simulink library "usask_tlm_lib"  (R2017b)
settings: Solver=ode45  StartTime=0.0  StopTime=10.0  RelTol=1e-3
undefined symbols (not defined in the file or in its folder): B, beta, d, K, L, lambda_1, m_E, m_G, mE_1, mE_2, mG_1, mG_2, nu, r1, r2, rho, T, Zc, Zc_1, Zc_2
libraries: usask_tlm_lib x6, transmission_lines x2
(part 2 of 4)

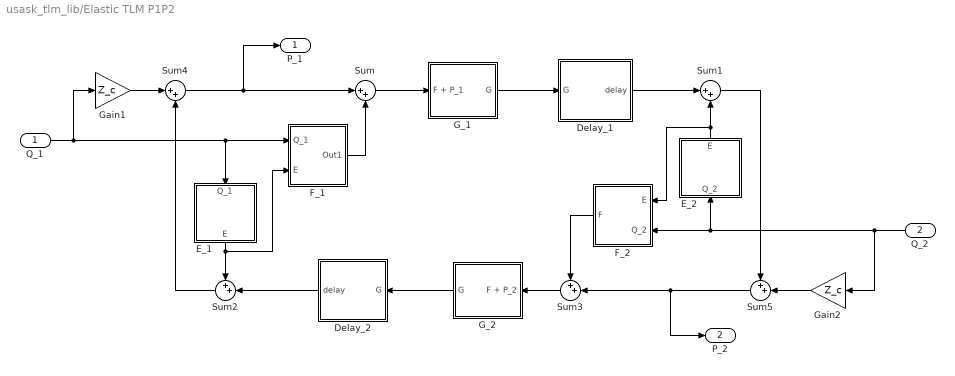
== system usask_tlm_lib/Elastic TLM P1P2 ==
  Q_1 : Inport
  Q_2 : Inport  Port=2
  "  Delay_2 " : Subsystem
      mask Display: disp('\fontname{Times New Roman}\ite^{-j\omegaT}', 'texmode', 'on')
  "Delay_1 " : Subsystem
      mask Display: disp('\fontname{Times New Roman}\ite^{-j\omegaT}', 'texmode', 'on')
  E_1 : Subsystem
      mask Display: disp('\fontname{Times New Roman}\fontsize{30}\itE', 'texmode', 'on')
  E_2 : Subsystem
      mask Display: disp('\fontname{Times New Roman}\fontsize{30}\itE', 'texmode', 'on')
  F_1 : Subsystem
      mask Display: disp('\fontname{Times New Roman}\fontsize{30}\itF', 'texmode', 'on')
  F_2 : Subsystem
      mask Display: disp('\fontname{Times New Roman}\fontsize{30}\itF', 'texmode', 'on')
  G_1 : Subsystem
      mask Display: disp('\fontname{Times New Roman}\fontsize{30}\itG', 'texmode', 'on')
  G_2 : Subsystem
      mask Display: disp('\fontname{Times New Roman}\fontsize{30}\itG', 'texmode', 'on')
  Gain1 : Gain  Gain=Z_c
  Gain2 : Gain  Gain=Z_c
  Sum : Sum  Inputs=|++
  Sum1 : Sum  Inputs=|++
  Sum2 : Sum  Inputs=++|
  Sum3 : Sum  Inputs=++|
  Sum4 : Sum  Inputs=|++
  Sum5 : Sum  Inputs=++|
  P_1 : Outport
  P_2 : Outport  Port=2
  wires:
  Sum/1 -> G_1/1(F + P_1)
  G_1/1(G) -> "Delay_1 "/1(G)
  E_2/1(E) -> Sum1/2, F_2/1(E)
  E_1/1(E) -> F_1/2(E), Sum2/1
  G_2/1(G) -> "  Delay_2 "/1(G)
  Q_1/1 -> Gain1/1, F_1/1(Q_1), E_1/1(Q_1)
  Sum4/1 -> P_1/1, Sum/1
  Sum3/1 -> G_2/1(F + P_2)
  F_2/1(F) -> Sum3/1
  Sum2/1 -> Sum4/2
  "Delay_1 "/1(delay) -> Sum1/1
  "  Delay_2 "/1(delay) -> Sum2/2
  Q_2/1 -> Gain2/1, F_2/2(Q_2), E_2/1(Q_2)
  Gain1/1 -> Sum4/1
  F_1/1(Out1) -> Sum/2
  Sum1/1 -> Sum5/1
  Gain2/1 -> Sum5/2
  Sum5/1 -> P_2/1, Sum3/2

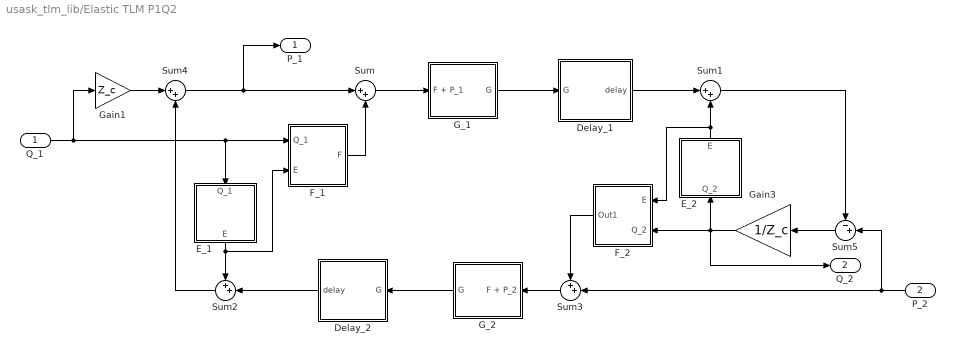
== system usask_tlm_lib/Elastic TLM P1Q2 ==
  Q_1 : Inport
  P_2 : Inport  Port=2
  "  Delay_2 " : Subsystem
      mask Display: disp('\fontname{Times New Roman}\ite^{-j\omegaT}', 'texmode', 'on')
  "Delay_1 " : Subsystem
      mask Display: disp('\fontname{Times New Roman}\ite^{-j\omegaT}', 'texmode', 'on')
  E_1 : Subsystem
      mask Display: disp('\fontname{Times New Roman}\fontsize{30}\itE', 'texmode', 'on')
  E_2 : Subsystem
      mask Display: disp('\fontname{Times New Roman}\fontsize{30}\itE', 'texmode', 'on')
  F_1 : Subsystem
      mask Display: disp('\fontname{Times New Roman}\fontsize{30}\itF', 'texmode', 'on')
  F_2 : Subsystem
      mask Display: disp('\fontname{Times New Roman}\fontsize{30}\itF', 'texmode', 'on')
  G_1 : Subsystem
      mask Display: disp('\fontname{Times New Roman}\fontsize{30}\itG', 'texmode', 'on')
  G_2 : Subsystem
      mask Display: disp('\fontname{Times New Roman}\fontsize{30}\itG', 'texmode', 'on')
  Gain1 : Gain  Gain=Z_c
  Gain3 : Gain  Gain=1/Z_c
  Sum : Sum  Inputs=|++
  Sum1 : Sum  Inputs=|++
  Sum2 : Sum  Inputs=++|
  Sum3 : Sum  Inputs=++|
  Sum4 : Sum  Inputs=|++
  Sum5 : Sum  Inputs=-+|
  P_1 : Outport
  Q_2 : Outport  Port=2
  wires:
  Sum/1 -> G_1/1(F + P_1)
  G_1/1(G) -> "Delay_1 "/1(G)
  E_2/1(E) -> Sum1/2, F_2/1(E)
  E_1/1(E) -> F_1/2(E), Sum2/1
  G_2/1(G) -> "  Delay_2 "/1(G)
  Q_1/1 -> Gain1/1, F_1/1(Q_1), E_1/1(Q_1)
  Sum4/1 -> P_1/1, Sum/1
  Sum3/1 -> G_2/1(F + P_2)
  F_2/1(Out1) -> Sum3/1
  Sum2/1 -> Sum4/2
  Sum1/1 -> Sum5/1
  P_2/1 -> Sum5/2, Sum3/2
  "Delay_1 "/1(delay) -> Sum1/1
  "  Delay_2 "/1(delay) -> Sum2/2
  Gain3/1 -> F_2/2(Q_2), E_2/1(Q_2), Q_2/1
  Gain1/1 -> Sum4/1
  Sum5/1 -> Gain3/1
  F_1/1(F) -> Sum/2

== system usask_tlm_lib/Elastic TLM Q1P2 ==
  P_1 : Inport
  Q_2 : Inport  Port=2
  "  Delay_2 " : Subsystem
      mask Display: disp('\fontname{Times New Roman}\ite^{-j\omegaT}', 'texmode', 'on')
  "Delay_1 " : Subsystem
      mask Display: disp('\fontname{Times New Roman}\ite^{-j\omegaT}', 'texmode', 'on')
  E_1 : Subsystem
      mask Display: disp('\fontname{Times New Roman}\fontsize{30}\itE', 'texmode', 'on')
  E_2 : Subsystem
      mask Display: disp('\fontname{Times New Roman}\fontsize{30}\itE', 'texmode', 'on')
  F_1 : Subsystem
      mask Display: disp('\fontname{Times New Roman}\fontsize{30}\itF', 'texmode', 'on')
  F_2 : Subsystem
      mask Display: disp('\fontname{Times New Roman}\fontsize{30}\itF', 'texmode', 'on')
  G_1 : Subsystem
      mask Display: disp('\fontname{Times New Roman}\fontsize{30}\itG', 'texmode', 'on')
  G_2 : Subsystem
      mask Display: disp('\fontname{Times New Roman}\fontsize{30}\itG', 'texmode', 'on')
  Gain1 : Gain  Gain=Z_c
  Gain2 : Gain  Gain=1/Z_c
  Sum : Sum  Inputs=|++
  Sum1 : Sum  Inputs=|++
  Sum2 : Sum  Inputs=++|
  Sum3 : Sum  Inputs=++|
  Sum4 : Sum  Inputs=++|
  Sum6 : Sum  Inputs=|+-
  Q_1 : Outport
  P_2 : Outport  Port=2
  wires:
  Sum/1 -> G_1/1(F + P_1)
  G_1/1(G) -> "Delay_1 "/1(G)
  E_2/1(E) -> Sum1/2, F_2/1(E)
  E_1/1(E) -> F_1/2(E), Sum2/1
  G_2/1(G) -> "  Delay_2 "/1(G)
  P_1/1 -> Sum6/1, Sum/1
  Sum3/1 -> G_2/1(F + P_2)
  F_2/1(Out1) -> Sum3/1
  "Delay_1 "/1(delay) -> Sum1/1
  "  Delay_2 "/1(delay) -> Sum2/2
  Q_2/1 -> Gain1/1, F_2/2(Q_2), E_2/1(Q_2)
  F_1/1(F) -> Sum/2
  Sum6/1 -> Gain2/1
  Gain2/1 -> Q_1/1, F_1/1(Q_1), E_1/1(Q_1)
  Sum2/1 -> Sum6/2
  Sum1/1 -> Sum4/1
  Sum4/1 -> P_2/1, Sum3/2
  Gain1/1 -> Sum4/2

== system usask_tlm_lib/Elastic TLM Q1Q2 ==
  P_1 : Inport
  P_2 : Inport  Port=2
  "  Delay_2 " : Subsystem
      mask Display: disp('\fontname{Times New Roman}\ite^{-j\omegaT}', 'texmode', 'on')
  "Delay_1 " : Subsystem
      mask Display: disp('\fontname{Times New Roman}\ite^{-j\omegaT}', 'texmode', 'on')
  E_1 : Subsystem
      mask Display: disp('\fontname{Times New Roman}\fontsize{30}\itE', 'texmode', 'on')
  E_2 : Subsystem
      mask Display: disp('\fontname{Times New Roman}\fontsize{30}\itE', 'texmode', 'on')
  F_1 : Subsystem
      mask Display: disp('\fontname{Times New Roman}\fontsize{30}\itF', 'texmode', 'on')
  F_2 : Subsystem
      mask Display: disp('\fontname{Times New Roman}\fontsize{30}\itF', 'texmode', 'on')
  G_1 : Subsystem
      mask Display: disp('\fontname{Times New Roman}\fontsize{30}\itG', 'texmode', 'on')
  G_2 : Subsystem
      mask Display: disp('\fontname{Times New Roman}\fontsize{30}\itG', 'texmode', 'on')
  Gain2 : Gain  Gain=1/Z_c
  Gain3 : Gain  Gain=1/Z_c
  Sum : Sum  Inputs=|++
  Sum1 : Sum  Inputs=|++
  Sum2 : Sum  Inputs=++|
  Sum3 : Sum  Inputs=++|
  Sum5 : Sum  Inputs=-+|
  Sum6 : Sum  Inputs=|+-
  Q_1 : Outport
  Q_2 : Outport  Port=2
  wires:
  Sum/1 -> G_1/1(F + P_1)
  G_1/1(G) -> "Delay_1 "/1(G)
  E_2/1(E) -> Sum1/2, F_2/1(E)
  E_1/1(E) -> F_1/2(E), Sum2/1
  G_2/1(G) -> "  Delay_2 "/1(G)
  Sum3/1 -> G_2/1(F + P_2)
  F_2/1(F) -> Sum3/1
  Sum1/1 -> Sum5/1
  P_2/1 -> Sum5/2, Sum3/2
  "Delay_1 "/1(delay) -> Sum1/1
  "  Delay_2 "/1(delay) -> Sum2/2
  Gain3/1 -> F_2/2(Q_2), E_2/1(Q_2), Q_2/1
  Sum5/1 -> Gain3/1
  F_1/1(F) -> Sum/2
  P_1/1 -> Sum6/1, Sum/1
  Sum6/1 -> Gain2/1
  Gain2/1 -> Q_1/1, F_1/1(Q_1), E_1/1(Q_1)
  Sum2/1 -> Sum6/2

== system usask_tlm_lib/Internal Blocks ==
  Tapered TLM Base : Subsystem  mask(Tapered Hydraulic Transmission Line (TLM)){Zc_1=Zc_1, Zc_2=Zc_2, beta=beta, T=T, lambda_1=lambda_1}
      mask help:
      | This model implements the transmission line model in Wiens and ven der Buhs (2018).
      |
      | This model assumes laminar flow in a rigid-walled tube with a linear taper in radius between the two ports. It assumes constant bulk modulus (no cavitation or entrined air effects) and includes frequency-dependent friction effects.
      |
      | Positive flows are directed into either port.
      |
      | This model also assumes zero initial conditions
      |
      | Reference:
      | Travis Wiens and Jeremy vsn der Buhs. In Improved Transmission Line Model for Dynamic Laminar Flow Through Tapered Tubes. Proceedings of the Bath/ASME Symposium on Fluid Power and Motion Control, Bath, 2018
      mask init:
      | lambda_2=1/lambda_1;
      | 
      | R=Zc_1*beta*8*(3/(1+lambda_1+lambda_1^2));%laminar resistance
      | 
      | k=6; % Number of weighting factors
      | 
      | % Grab optimized weighting factors and parameters. Please see paper for
      | % more detail on how these parameters were found.
      | [ mE_1, mG_1, tau_1, K_diff1, K_mean1 ] = interpolateTLMparamsFIR( beta, lambda_1, k);
      | [ mE_2, mG_2, tau_2, K_diff2, K_mean2 ] = interpolateTLMparamsFIR( beta, lambda_2, k);
      | 
      | %Todo: fix error checkings
      | % if isnan(mE_1(1)) || isnan(mG_1(1)) || isnan(tau_1) ||isnan(mE_2(1)) || isnan(mG_2(1)) || isnan(tau_2)
      | %     error('The parameters you have entered are outside the working range of this model. Weighting factors cannot be found')
      | % end
      | 
      | T_1 = tau_1*T; % Modified wave propagation time (s), Equation (18)
      | T_2 = tau_2*T; % Modified wave propagation time (s), Equation (18)
      | 
      | n=nan(1,k); % Weighting factor initialization
      | n(1)=0.3/(1+3*beta);
      | for i=2:k
      |     n(i)=n(i-1)*3; 
      | end
      | 
      | % H 
      | H_1DC=K_mean1*(1/lambda_1.^2 -1)/(8*beta*3/(1+lambda_1+lambda_1^2)+1/lambda_1^2+1);
      | H_2DC=K_mean2*(1/lambda_2.^2 -1)/(8*beta*3/(1+lambda_2+lambda_2^2)+1/lambda_2^2+1);
      | 
      | H_1mean=H_1DC/(2*T_1);
      | H_2mean=H_2DC/(2*T_2);
      | 
      | H_1a=K_diff1*H_1mean;
      | H_1b=(2-K_diff1)*H_1mean;
      | 
      | H_2a=K_diff2*H_2mean;
      | H_2b=(2-K_diff2)*H_2mean;
      | 
      | 
      | % E
      | E_1DC=Zc_1*sum(mE_1./n);
      | E_2DC=Zc_2*sum(mE_2./n);
      | 
      | b_1=1-8*beta/(E_1DC/Zc_1);
      | b_2=1-8*beta/(E_2DC/Zc_2);
      | 
      | % F
      | F_1DC=Zc_1+b_1*E_1DC;
      | F_2DC=Zc_2+b_2*E_2DC;
      | 
      | F_k1=((1-H_1DC)*(E_2DC+Zc_2-R)+H_2DC*(E_1DC+Zc_1))/(1-H_1DC-H_2DC)/F_1DC
      | F_k2=((1-H_2DC)*(E_1DC+Zc_1-R)+H_1DC*(E_2DC+Zc_2))/(1-H_2DC-H_1DC)/F_2DC
      | 
      | %Error Checking
      | % load TaperedTLMAcceptableErrorContour.mat
      | % IN = inpolygon(lambda_1,beta,lambda_poly,beta_poly);
      | % if ~IN
      | %     warning('Dissipaton number (beta) and taper ratio (lambda) combination are outside the recommended range')
      | % end
      | %warning('need to reinstate polygon error checking')
      | 
      | 
      | 
      | 
      | %% End of initialization
      mask DialogControl DescGroupVar Prompt: Tapered Hydraulic Transmission Line (TLM)
  Tapered TLM Segment : Subsystem  mask(Tapered Hydraulic Transmission Line (TLM)){Zc_1=Zc(2), Zc_2=Zc(3), beta=beta(2), T=T(2), lambda_1=lambda_1(2)}
      mask help:
      | This model implements the transmission line model in Wiens and ven der Buhs (2018).
      |
      | This model assumes a rigid-walled tube with a linear taper in radius between the two ports. It assumes constant bulk modulus (no cavitation or entrined air effects) and includes frequency-dependent friction effects.
      |
      | Positive flows are directed into either port.
      |
      | This model also assumes zero initial conditions
      |
      | Reference:
      | Travis Wiens and Jeremy vsn der Buhs. In Improved Transmission Line Model for Dynamic Laminar Flow Through Tapered Tubes. Proceedings of the Bath/ASME Symposium on Fluid Power and Motion Control, Bath, 2018
      mask init:
      | lambda_2=1/lambda_1;
      | 
      | R=Zc_1*beta*8*(3/(1+lambda_1+lambda_1^2));%laminar resistance
      | 
      | k=6; % Number of weighting factors
      | 
      | % Grab optimized weighting factors and parameters. Please see paper for
      | % more detail on how these parameters were found.
      | [ mE_1, mG_1, tau_1, K_diff1, K_mean1 ] = interpolateTLMparamsFIR( beta, lambda_1, k);
      | [ mE_2, mG_2, tau_2, K_diff2, K_mean2 ] = interpolateTLMparamsFIR( beta, lambda_2, k);
      | 
      | %Todo: fix error checkings
      | % if isnan(mE_1(1)) || isnan(mG_1(1)) || isnan(tau_1) ||isnan(mE_2(1)) || isnan(mG_2(1)) || isnan(tau_2)
      | %     error('The parameters you have entered are outside the working range of this model. Weighting factors cannot be found')
      | % end
      | 
      | T_1 = tau_1*T; % Modified wave propagation time (s), Equation (18)
      | T_2 = tau_2*T; % Modified wave propagation time (s), Equation (18)
      | 
      | n=nan(1,k); % Weighting factor initialization
      | n(1)=0.3/(1+3*beta);
      | for i=2:k
      |     n(i)=n(i-1)*3; 
      | end
      | 
      | % H 
      | H_1DC=K_mean1*(1/lambda_1.^2 -1)/(8*beta*3/(1+lambda_1+lambda_1^2)+1/lambda_1^2+1);
      | H_2DC=K_mean2*(1/lambda_2.^2 -1)/(8*beta*3/(1+lambda_2+lambda_2^2)+1/lambda_2^2+1);
      | 
      | C_1mean=H_1DC/(2*T_1);
      | C_2mean=H_2DC/(2*T_2);
      | 
      | % C_1mean=H_1DC;
      | % C_2mean=H_2DC;
      | 
      | H_1a=K_diff1*C_1mean;
      | H_1b=(2-K_diff1)*C_1mean;
      | 
      | H_2a=K_diff2*C_2mean;
      | H_2b=(2-K_diff2)*C_2mean;
      | 
      | 
      | %N_H=100;%make this a parameter
      | 
      | %H_1=[linspace(H_1a,H_1b,N_H)]*(2*T_1)./(N_H);
      | %H_2=[linspace(H_2a,H_2b,N_H)]*(2*T_2)./(N_H);
      | 
      | % E
      | E_1DC=Zc_1*sum(mE_1./n);
      | E_2DC=Zc_2*sum(mE_2./n);
      | 
      | b_1=1-8*beta/(E_1DC/Zc_1);% eq (16)
      | b_2=1-8*beta/(E_2DC/Zc_2);% eq (16)
      | 
      | % F
      | F_1DC=Zc_1+b_1*E_1DC;
      | F_2DC=Zc_2+b_2*E_2DC;
      | 
      | F_k1=((1-H_1DC)*(E_2DC+Zc_2-R)+H_2DC*(E_1DC+Zc_1))/(1-H_1DC-H_2DC)/F_1DC
      | F_k2=((1-H_2DC)*(E_1DC+Zc_1-R)+H_1DC*(E_2DC+Zc_2))/(1-H_2DC-H_1DC)/F_2DC
      | 
      | %Error Checking
      | % load TaperedTLMAcceptableErrorContour.mat
      | % IN = inpolygon(lambda_1,beta,lambda_poly,beta_poly);
      | % if ~IN
      | %     warning('Dissipaton number (beta) and taper ratio (lambda) combination are outside the recommended range')
      | % end
      | warning('need to reinstate polygon error checking')
      | 
      | 
      | 
      | 
      | %% End of initialization
      mask DialogControl DescGroupVar Prompt: Tapered Hydraulic Transmission Line (TLM)

== system usask_tlm_lib/TLM Johnston P1P2 ==
  Q1 : Inport
  Q2 : Inport  Port=2
  E1 : transmission_lines/TLM Krus P1P2/E1
  E2 : Subsystem
  F1 : transmission_lines/TLM Krus P1P2/F1
  F2 : Subsystem
  G1 : Subsystem
  G2 : Subsystem
  Gain : Gain  Gain=Zc
  Gain1 : Gain  Gain=Zc
  Sum : Sum  Inputs=|++
  Sum1 : Sum  Inputs=++|
  Sum2 : Sum  Inputs=++|
  Sum3 : Sum  Inputs=|++
  Sum4 : Sum  Inputs=|++
  Sum5 : Sum  Inputs=++|
  Transport Delay1 : TransportDelay  DelayTime=T
  Transport Delay2 : TransportDelay  DelayTime=T
  P1 : Outport
  P2 : Outport  Port=2
  wires:
  Sum3/1 -> Sum5/1  "C2"
  G1/1(Out) -> Transport Delay1/1
  E2/1(Out) -> Sum3/2
  Sum5/1 -> Sum2/2, P2/1  "P2"
  Sum2/1 -> G2/1(In)
  F2/1(Out) -> Sum2/1
  Q2/1 -> F2/1(In), E2/1(In), Gain1/1  "Q2"
  Transport Delay1/1 -> Sum3/1
  Gain1/1 -> Sum5/2
  Sum/1 -> G1/1(In)
  Transport Delay2/1 -> Sum1/2
  Sum1/1 -> Sum4/1  "C1"
  F1/1 -> Sum/2
  E1/1 -> Sum1/1
  G2/1(Out) -> Transport Delay2/1
  Q1/1 -> Gain/1, F1/1, E1/1  "Q1"
  Sum4/1 -> P1/1, Sum/1  "P1"
  Gain/1 -> Sum4/2

== system usask_tlm_lib/TLM Johnston P1Q2 ==
  Q1 : Inport
  P2 : Inport  Port=2
  Ea : Subsystem
  Eb : Subsystem
  Fa : Subsystem
  Fb : Subsystem
  Ga : Subsystem
  Gain : Gain  Gain=Zc
  Gain1 : Gain  Gain=1/Zc
  Gb : Subsystem
  Sum : Sum  Inputs=|++
  Sum1 : Sum  Inputs=++|
  Sum2 : Sum  Inputs=++|
  Sum3 : Sum  Inputs=|++
  Sum4 : Sum  Inputs=|++
  Sum5 : Sum  Inputs=-+|
  Transport Delay1 : TransportDelay  DelayTime=T
  Transport Delay2 : TransportDelay  DelayTime=T
  P1 : Outport
  Q2 : Outport  Port=2
  wires:
  Sum4/1 -> P1/1, Sum/1  "P1"
  Sum/1 -> Ga/1(In)
  Transport Delay2/1 -> Sum3/1
  Gain/1 -> Sum4/1
  Sum5/1 -> Gain1/1
  Transport Delay1/1 -> Sum1/2
  Q1/1 -> Gain/1, Ea/1(In), Fa/1(In)
  Sum1/1 -> Sum4/2
  Fa/1(Out) -> Sum/2
  Gain1/1 -> Q2/1, Eb/1(In), Fb/1(In)  "Q2"
  Fb/1(Out) -> Sum2/1
  Sum2/1 -> Gb/1(In)
  Ea/1(Out) -> Sum1/1
  Gb/1(Out) -> Transport Delay1/1
  P2/1 -> Sum5/2, Sum2/2
  Eb/1(Out) -> Sum3/2
  Ga/1(Out) -> Transport Delay2/1
  Sum3/1 -> Sum5/1  "C2"

== system usask_tlm_lib/TLM Johnston Q1P2 ==
  P1 : Inport
  Q2 : Inport  Port=2
  Ea : Subsystem
  Eb : Subsystem
  Fa : Subsystem
  Fb : Subsystem
  Ga : Subsystem
  Gain : Gain  Gain=1/Zc
  Gain1 : Gain  Gain=Zc
  Gb : Subsystem
  Sum : Sum  Inputs=|++
  Sum1 : Sum  Inputs=++|
  Sum2 : Sum  Inputs=++|
  Sum3 : Sum  Inputs=|++
  Sum4 : Sum  Inputs=|+-
  Sum5 : Sum  Inputs=++|
  Transport Delay1 : TransportDelay  DelayTime=T
  Transport Delay2 : TransportDelay  DelayTime=T
  Q1 : Outport
  P2 : Outport  Port=2
  wires:
  Gain1/1 -> Sum5/2
  P1/1 -> Sum4/1, Sum/1  "P1"
  Sum/1 -> Ga/1(In)
  Transport Delay2/1 -> Sum3/1
  Transport Delay1/1 -> Sum1/2
  Gain/1 -> Q1/1, Ea/1(In), Fa/1(In)  "Q1"
  Sum1/1 -> Sum4/2  "C1"
  Fa/1(Out) -> Sum/2
  Q2/1 -> Gain1/1, Eb/1(In), Fb/1(In)  "Q2"
  Fb/1(Out) -> Sum2/1
  Sum2/1 -> Gb/1(In)
  Ea/1(Out) -> Sum1/1
  Gb/1(Out) -> Transport Delay1/1
  Sum5/1 -> P2/1, Sum2/2  "P2"
  Eb/1(Out) -> Sum3/2
  Ga/1(Out) -> Transport Delay2/1
  Sum3/1 -> Sum5/1  "C2"
  Sum4/1 -> Gain/1

== system usask_tlm_lib/TLM Johnston Q1Q2 ==
  P1 : Inport
  P2 : Inport  Port=2
  Ea : Subsystem
  Eb : Subsystem
  Fa : Subsystem
  Fb : Subsystem
  Ga : Subsystem
  Gain : Gain  Gain=1/Zc
  Gain1 : Gain  Gain=1/Zc
  Gb : Subsystem
  Sum : Sum  Inputs=|++
  Sum1 : Sum  Inputs=++|
  Sum2 : Sum  Inputs=++|
  Sum3 : Sum  Inputs=|++
  Sum4 : Sum  Inputs=|+-
  Sum5 : Sum  Inputs=-+|
  Transport Delay1 : TransportDelay  DelayTime=T
  Transport Delay2 : TransportDelay  DelayTime=T
  Q1 : Outport
  Q2 : Outport  Port=2
  wires:
  P1/1 -> Sum4/1, Sum/1  "P1"
  Sum/1 -> Ga/1(In)
  Transport Delay2/1 -> Sum3/1
  Sum5/1 -> Gain1/1
  Transport Delay1/1 -> Sum1/2
  Gain/1 -> Q1/1, Ea/1(In), Fa/1(In)  "Q1"
  Sum1/1 -> Sum4/2  "C1"
  Fa/1(Out) -> Sum/2
  Gain1/1 -> Q2/1, Eb/1(In), Fb/1(In)  "Q2"
  Fb/1(Out) -> Sum2/1
  Sum2/1 -> Gb/1(In)
  Ea/1(Out) -> Sum1/1
  Gb/1(Out) -> Transport Delay1/1
  P2/1 -> Sum5/2, Sum2/2
  Eb/1(Out) -> Sum3/2
  Ga/1(Out) -> Transport Delay2/1
  Sum3/1 -> Sum5/1  "C2"
  Sum4/1 -> Gain/1

== system usask_tlm_lib/TLM Krus P1P2 ==
  Q1 : Inport
  Q2 : Inport  Port=2
  E1 : Subsystem
  E2 : Subsystem
  F1 : Subsystem
  F2 : Subsystem
  G1 : Subsystem
  G2 : Subsystem
  Gain : Gain  Gain=Zc
  Gain1 : Gain  Gain=Zc
  Sum : Sum  Inputs=|++
  Sum1 : Sum  Inputs=++|
  Sum2 : Sum  Inputs=++|
  Sum3 : Sum  Inputs=|++
  Sum4 : Sum  Inputs=|++
  Sum5 : Sum  Inputs=++|
  Transport Delay1 : TransportDelay  DelayTime=T
  Transport Delay2 : TransportDelay  DelayTime=T
  P1 : Outport
  P2 : Outport  Port=2
  wires:
  Gain/1 -> Sum4/2
  Sum4/1 -> Sum/1, P1/1  "P1"
  Q1/1 -> E1/1(In), F1/1(In), Gain/1  "Q1"
  Sum3/1 -> Sum5/1  "C2"
  Sum5/1 -> P2/1, Sum2/2  "P2"
  Q2/1 -> E2/1(In), F2/1(In), Gain1/1  "Q2"
  Gain1/1 -> Sum5/2
  G1/1(Out) -> Transport Delay2/1
  E2/1(Out) -> Sum3/2
  G2/1(Out) -> Transport Delay1/1
  E1/1(Out) -> Sum1/1
  Sum2/1 -> G2/1(In)
  F2/1(Out) -> Sum2/1
  F1/1(Out) -> Sum/2
  Sum1/1 -> Sum4/1  "C1"
  Transport Delay1/1 -> Sum1/2
  Transport Delay2/1 -> Sum3/1
  Sum/1 -> G1/1(In)

== system usask_tlm_lib/TLM Krus P1Q2 ==
  Q1 : Inport
  P2 : Inport  Port=2
  E1 : Subsystem
  E2 : Subsystem
  F1 : Subsystem
  F2 : Subsystem
  G1 : Subsystem
  G2 : Subsystem
  Gain : Gain  Gain=Zc
  Gain1 : Gain  Gain=1/Zc
  Sum : Sum  Inputs=|++
  Sum1 : Sum  Inputs=++|
  Sum2 : Sum  Inputs=++|
  Sum3 : Sum  Inputs=|++
  Sum4 : Sum  Inputs=|++
  Sum5 : Sum  Inputs=-+|
  Transport Delay1 : TransportDelay  DelayTime=T
  Transport Delay2 : TransportDelay  DelayTime=T
  P1 : Outport
  Q2 : Outport  Port=2
  wires:
  Sum4/1 -> P1/1, Sum/1  "P1"
  Sum/1 -> G1/1(In)
  Transport Delay2/1 -> Sum3/1
  Gain/1 -> Sum4/1
  Sum5/1 -> Gain1/1
  Transport Delay1/1 -> Sum1/2
  Q1/1 -> Gain/1, E1/1(In), F1/1(In)
  Sum1/1 -> Sum4/2
  F1/1(Out) -> Sum/2
  Gain1/1 -> Q2/1, E2/1(In), F2/1(In)  "Q2"
  F2/1(Out) -> Sum2/1
  Sum2/1 -> G2/1(In)
  E1/1(Out) -> Sum1/1
  G2/1(Out) -> Transport Delay1/1
  P2/1 -> Sum5/2, Sum2/2
  E2/1(Out) -> Sum3/2
  G1/1(Out) -> Transport Delay2/1
  Sum3/1 -> Sum5/1  "C2"

== system usask_tlm_lib/TLM Krus Q1P2 ==
  P1 : Inport
  Q2 : Inport  Port=2
  E1 : Subsystem
  E2 : Subsystem
  F1 : Subsystem
  F2 : Subsystem
  G1 : Subsystem
  G2 : Subsystem
  Gain : Gain  Gain=1/Zc
  Gain1 : Gain  Gain=Zc
  Sum : Sum  Inputs=|++
  Sum1 : Sum  Inputs=++|
  Sum2 : Sum  Inputs=++|
  Sum3 : Sum  Inputs=|++
  Sum4 : Sum  Inputs=|+-
  Sum5 : Sum  Inputs=++|
  Transport Delay1 : TransportDelay  DelayTime=T
  Transport Delay2 : TransportDelay  DelayTime=T
  Q1 : Outport
  P2 : Outport  Port=2
  wires:
  Sum3/1 -> Sum5/1  "C2"
  Sum5/1 -> P2/1, Sum2/2  "P2"
  Q2/1 -> E2/1(In), F2/1(In), Gain1/1  "Q2"
  Gain1/1 -> Sum5/2
  Sum4/1 -> Gain/1
  G1/1(Out) -> Transport Delay2/1
  E2/1(Out) -> Sum3/2
  G2/1(Out) -> Transport Delay1/1
  E1/1(Out) -> Sum1/1
  Sum2/1 -> G2/1(In)
  F2/1(Out) -> Sum2/1
  F1/1(Out) -> Sum/2
  Sum1/1 -> Sum4/2  "C1"
  Gain/1 -> Q1/1, E1/1(In), F1/1(In)  "Q1"
  Transport Delay1/1 -> Sum1/2
  Transport Delay2/1 -> Sum3/1
  Sum/1 -> G1/1(In)
  P1/1 -> Sum4/1, Sum/1  "P1"

== system usask_tlm_lib/TLM Krus Q1Q2 ==
  P1 : Inport
  P2 : Inport  Port=2
  E1 : Subsystem
  E2 : Subsystem
  F1 : Subsystem
  F2 : Subsystem
  G1 : Subsystem
  G2 : Subsystem
  Gain : Gain  Gain=1/Zc
  Gain1 : Gain  Gain=1/Zc
  Sum : Sum  Inputs=|++
  Sum1 : Sum  Inputs=++|
  Sum2 : Sum  Inputs=++|
  Sum3 : Sum  Inputs=|++
  Sum4 : Sum  Inputs=|+-
  Sum5 : Sum  Inputs=-+|
  Transport Delay1 : TransportDelay  DelayTime=T
  Transport Delay2 : TransportDelay  DelayTime=T
  Q1 : Outport
  Q2 : Outport  Port=2
  wires:
  Sum4/1 -> Gain/1
  Sum3/1 -> Sum5/1  "C2"
  G1/1(Out) -> Transport Delay2/1
  E2/1(Out) -> Sum3/2
  P2/1 -> Sum2/2, Sum5/2
  G2/1(Out) -> Transport Delay1/1
  E1/1(Out) -> Sum1/1
  Sum2/1 -> G2/1(In)
  F2/1(Out) -> Sum2/1
  Gain1/1 -> F2/1(In), E2/1(In), Q2/1  "Q2"
  F1/1(Out) -> Sum/2
  Sum1/1 -> Sum4/2  "C1"
  Gain/1 -> Q1/1, E1/1(In), F1/1(In)  "Q1"
  Transport Delay1/1 -> Sum1/2
  Sum5/1 -> Gain1/1
  Transport Delay2/1 -> Sum3/1
  Sum/1 -> G1/1(In)
  P1/1 -> Sum4/1, Sum/1  "P1"

== system usask_tlm_lib/Tapered Elastic TLM P1P2 ==
  Q_1 : Inport
  Q_2 : Inport  Port=2
  "  Delay_2 " : Subsystem
      mask Display: disp('\fontname{Times New Roman}\ite^{-j\omegaT}', 'texmode', 'on')
  "Delay_1 " : Subsystem
      mask Display: disp('\fontname{Times New Roman}\ite^{-j\omegaT}', 'texmode', 'on')
  E_1 : Subsystem
      mask Display: disp('\fontname{Times New Roman}\fontsize{30}\itE', 'texmode', 'on')
  E_2 : Subsystem
      mask Display: disp('\fontname{Times New Roman}\fontsize{30}\itE', 'texmode', 'on')
  F_1 : Subsystem
      mask Display: disp('\fontname{Times New Roman}\fontsize{30}\itF', 'texmode', 'on')
  F_2 : Subsystem
      mask Display: disp('\fontname{Times New Roman}\fontsize{30}\itF', 'texmode', 'on')
  G_1 : Subsystem
      mask Display: disp('\fontname{Times New Roman}\fontsize{30}\itG', 'texmode', 'on')
  G_2 : Subsystem
      mask Display: disp('\fontname{Times New Roman}\fontsize{30}\itG', 'texmode', 'on')
  Gain1 : Gain  Gain=Z_c
  Gain2 : Gain  Gain=Z_c
  Sum : Sum  Inputs=|++
  Sum1 : Sum  Inputs=|++
  Sum2 : Sum  Inputs=++|
  Sum3 : Sum  Inputs=++|
  Sum4 : Sum  Inputs=|++
  Sum5 : Sum  Inputs=++|
  P_1 : Outport
  P_2 : Outport  Port=2
  wires:
  Sum/1 -> G_1/1(F + P_1)
  G_1/1(G) -> "Delay_1 "/1(G)
  E_2/1(E) -> Sum1/2, F_2/1(E)
  E_1/1(E) -> F_1/2(E), Sum2/1
  G_2/1(G) -> "  Delay_2 "/1(G)
  Q_1/1 -> Gain1/1, F_1/1(Q_1), E_1/1(Q_1)
  Sum4/1 -> P_1/1, Sum/1
  Sum3/1 -> G_2/1(F + P_2)
  F_2/1(F) -> Sum3/1
  Sum2/1 -> Sum4/2
  "Delay_1 "/1(delay) -> Sum1/1
  "  Delay_2 "/1(delay) -> Sum2/2
  Q_2/1 -> Gain2/1, F_2/2(Q_2), E_2/1(Q_2)
  Gain1/1 -> Sum4/1
  F_1/1(Out1) -> Sum/2
  Sum1/1 -> Sum5/1
  Gain2/1 -> Sum5/2
  Sum5/1 -> P_2/1, Sum3/2

== system usask_tlm_lib/Tapered Elastic TLM P1Q2 ==
  Q_1 : Inport
  P_2 : Inport  Port=2
  "  Delay_2 " : Subsystem
      mask Display: disp('\fontname{Times New Roman}\ite^{-j\omegaT}', 'texmode', 'on')
  "Delay_1 " : Subsystem
      mask Display: disp('\fontname{Times New Roman}\ite^{-j\omegaT}', 'texmode', 'on')
  E_1 : Subsystem
      mask Display: disp('\fontname{Times New Roman}\fontsize{30}\itE', 'texmode', 'on')
  E_2 : Subsystem
      mask Display: disp('\fontname{Times New Roman}\fontsize{30}\itE', 'texmode', 'on')
  F_1 : Subsystem
      mask Display: disp('\fontname{Times New Roman}\fontsize{30}\itF', 'texmode', 'on')
  F_2 : Subsystem
      mask Display: disp('\fontname{Times New Roman}\fontsize{30}\itF', 'texmode', 'on')
  G_1 : Subsystem
      mask Display: disp('\fontname{Times New Roman}\fontsize{30}\itG', 'texmode', 'on')
  G_2 : Subsystem
      mask Display: disp('\fontname{Times New Roman}\fontsize{30}\itG', 'texmode', 'on')
  Gain1 : Gain  Gain=Z_c
  Gain3 : Gain  Gain=1/Z_c
  Sum : Sum  Inputs=|++
  Sum1 : Sum  Inputs=|++
  Sum2 : Sum  Inputs=++|
  Sum3 : Sum  Inputs=++|
  Sum4 : Sum  Inputs=|++
  Sum5 : Sum  Inputs=-+|
  P_1 : Outport
  Q_2 : Outport  Port=2
  wires:
  Sum/1 -> G_1/1(F + P_1)
  G_1/1(G) -> "Delay_1 "/1(G)
  E_2/1(E) -> Sum1/2, F_2/1(E)
  E_1/1(E) -> F_1/2(E), Sum2/1
  G_2/1(G) -> "  Delay_2 "/1(G)
  Q_1/1 -> Gain1/1, F_1/1(Q_1), E_1/1(Q_1)
  Sum4/1 -> P_1/1, Sum/1
  Sum3/1 -> G_2/1(F + P_2)
  F_2/1(Out1) -> Sum3/1
  Sum2/1 -> Sum4/2
  Sum1/1 -> Sum5/1
  P_2/1 -> Sum5/2, Sum3/2
  "Delay_1 "/1(delay) -> Sum1/1
  "  Delay_2 "/1(delay) -> Sum2/2
  Gain3/1 -> F_2/2(Q_2), E_2/1(Q_2), Q_2/1
  Gain1/1 -> Sum4/1
  Sum5/1 -> Gain3/1
  F_1/1(F) -> Sum/2

== system usask_tlm_lib/Tapered Elastic TLM Q1P2 ==
  P_1 : Inport
  Q_2 : Inport  Port=2
  "  Delay_2 " : Subsystem
      mask Display: disp('\fontname{Times New Roman}\ite^{-j\omegaT}', 'texmode', 'on')
  "Delay_1 " : Subsystem
      mask Display: disp('\fontname{Times New Roman}\ite^{-j\omegaT}', 'texmode', 'on')
  E_1 : Subsystem
      mask Display: disp('\fontname{Times New Roman}\fontsize{30}\itE', 'texmode', 'on')
  E_2 : Subsystem
      mask Display: disp('\fontname{Times New Roman}\fontsize{30}\itE', 'texmode', 'on')
  F_1 : Subsystem
      mask Display: disp('\fontname{Times New Roman}\fontsize{30}\itF', 'texmode', 'on')
  F_2 : Subsystem
      mask Display: disp('\fontname{Times New Roman}\fontsize{30}\itF', 'texmode', 'on')
  G_1 : Subsystem
      mask Display: disp('\fontname{Times New Roman}\fontsize{30}\itG', 'texmode', 'on')
  G_2 : Subsystem
      mask Display: disp('\fontname{Times New Roman}\fontsize{30}\itG', 'texmode', 'on')
  Gain1 : Gain  Gain=Z_c
  Gain2 : Gain  Gain=1/Z_c
  Sum : Sum  Inputs=|++
  Sum1 : Sum  Inputs=|++
  Sum2 : Sum  Inputs=++|
  Sum3 : Sum  Inputs=++|
  Sum4 : Sum  Inputs=++|
  Sum6 : Sum  Inputs=|+-
  Q_1 : Outport
  P_2 : Outport  Port=2
  wires:
  Sum/1 -> G_1/1(F + P_1)
  G_1/1(G) -> "Delay_1 "/1(G)
  E_2/1(E) -> Sum1/2, F_2/1(E)
  E_1/1(E) -> F_1/2(E), Sum2/1
  G_2/1(G) -> "  Delay_2 "/1(G)
  P_1/1 -> Sum6/1, Sum/1
  Sum3/1 -> G_2/1(F + P_2)
  F_2/1(Out1) -> Sum3/1
  "Delay_1 "/1(delay) -> Sum1/1
  "  Delay_2 "/1(delay) -> Sum2/2
  Q_2/1 -> Gain1/1, F_2/2(Q_2), E_2/1(Q_2)
  F_1/1(F) -> Sum/2
  Sum6/1 -> Gain2/1
  Gain2/1 -> Q_1/1, F_1/1(Q_1), E_1/1(Q_1)
  Sum2/1 -> Sum6/2
  Sum1/1 -> Sum4/1
  Sum4/1 -> P_2/1, Sum3/2
  Gain1/1 -> Sum4/2

== system usask_tlm_lib/Tapered Elastic TLM Q1Q2 ==
  P_1 : Inport
  P_2 : Inport  Port=2
  "  Delay_2 " : Subsystem
      mask Display: disp('\fontname{Times New Roman}\ite^{-j\omegaT}', 'texmode', 'on')
  "Delay_1 " : Subsystem
      mask Display: disp('\fontname{Times New Roman}\ite^{-j\omegaT}', 'texmode', 'on')
  E_1 : Subsystem
      mask Display: disp('\fontname{Times New Roman}\fontsize{30}\itE', 'texmode', 'on')
  E_2 : Subsystem
      mask Display: disp('\fontname{Times New Roman}\fontsize{30}\itE', 'texmode', 'on')
  F_1 : Subsystem
      mask Display: disp('\fontname{Times New Roman}\fontsize{30}\itF', 'texmode', 'on')
  F_2 : Subsystem
      mask Display: disp('\fontname{Times New Roman}\fontsize{30}\itF', 'texmode', 'on')
  G_1 : Subsystem
      mask Display: disp('\fontname{Times New Roman}\fontsize{30}\itG', 'texmode', 'on')
  G_2 : Subsystem
      mask Display: disp('\fontname{Times New Roman}\fontsize{30}\itG', 'texmode', 'on')
  Gain2 : Gain  Gain=1/Z_c
  Gain3 : Gain  Gain=1/Z_c
  Sum : Sum  Inputs=|++
  Sum1 : Sum  Inputs=|++
  Sum2 : Sum  Inputs=++|
  Sum3 : Sum  Inputs=++|
  Sum5 : Sum  Inputs=-+|
  Sum6 : Sum  Inputs=|+-
  Q_1 : Outport
  Q_2 : Outport  Port=2
  wires:
  Sum/1 -> G_1/1(F + P_1)
  G_1/1(G) -> "Delay_1 "/1(G)
  E_2/1(E) -> Sum1/2, F_2/1(E)
  E_1/1(E) -> F_1/2(E), Sum2/1
  G_2/1(G) -> "  Delay_2 "/1(G)
  Sum3/1 -> G_2/1(F + P_2)
  F_2/1(F) -> Sum3/1
  Sum1/1 -> Sum5/1
  P_2/1 -> Sum5/2, Sum3/2
  "Delay_1 "/1(delay) -> Sum1/1
  "  Delay_2 "/1(delay) -> Sum2/2
  Gain3/1 -> F_2/2(Q_2), E_2/1(Q_2), Q_2/1
  Sum5/1 -> Gain3/1
  F_1/1(F) -> Sum/2
  P_1/1 -> Sum6/1, Sum/1
  Sum6/1 -> Gain2/1
  Gain2/1 -> Q_1/1, F_1/1(Q_1), E_1/1(Q_1)
  Sum2/1 -> Sum6/2

== system usask_tlm_lib/Tapered FIR TLM P1P2 ==
  Q_1 : Inport
  Q_2 : Inport  Port=2
  Gain1 : Gain  Gain=Zc_2
  Gain2 : Gain  Gain=Zc_1
  Sum4 : Sum  Inputs=++|
  Sum6 : Sum  Inputs=++|
  Tapered TLM Base : usask_tlm_lib/Internal Blocks/Tapered TLM Base  Zc_1=Zc_1  Zc_2=Zc_2  beta=beta  T=T  lambda_1=lambda_1
      settings: SourceProductName=USask Transmission Line Model Library
  P_1 : Outport
  P_2 : Outport  Port=2
  wires:
  Tapered TLM Base/2 -> Sum4/1
  Gain1/1 -> Sum4/2
  Sum4/1 -> P_2/1, Tapered TLM Base/4
  Q_2/1 -> Gain1/1, Tapered TLM Base/3
  Tapered TLM Base/1 -> Sum6/1
  Sum6/1 -> Tapered TLM Base/1, P_1/1
  Q_1/1 -> Tapered TLM Base/2, Gain2/1
  Gain2/1 -> Sum6/2

== system usask_tlm_lib/Tapered FIR TLM P1Q2 ==
  Q_1 : Inport
  P_2 : Inport  Port=2
  Gain1 : Gain  Gain=1/Zc_2
  Gain2 : Gain  Gain=Zc_1
  Sum4 : Sum  Inputs=-+|
  Sum6 : Sum  Inputs=++|
  Tapered TLM Base : usask_tlm_lib/Internal Blocks/Tapered TLM Base  Zc_1=Zc_1  Zc_2=Zc_2  beta=beta  T=T  lambda_1=lambda_1
      settings: SourceProductName=USask Transmission Line Model Library
  P_1 : Outport
  Q_2 : Outport  Port=2
  wires:
  Gain1/1 -> Q_2/1, Tapered TLM Base/3
  Sum4/1 -> Gain1/1
  Tapered TLM Base/2 -> Sum4/1
  Tapered TLM Base/1 -> Sum6/1
  P_2/1 -> Tapered TLM Base/4, Sum4/2
  Sum6/1 -> P_1/1, Tapered TLM Base/1
  Gain2/1 -> Sum6/2
  Q_1/1 -> Tapered TLM Base/2, Gain2/1

== system usask_tlm_lib/Tapered FIR TLM Q1P2 ==
  P_1 : Inport
  Q_2 : Inport  Port=2
  Gain1 : Gain  Gain=Zc_2
  Gain2 : Gain  Gain=1/Zc_1
  Sum4 : Sum  Inputs=++|
  Sum6 : Sum  Inputs=|+-
  Tapered TLM Base : usask_tlm_lib/Internal Blocks/Tapered TLM Base  Zc_1=Zc_1  Zc_2=Zc_2  beta=beta  T=T  lambda_1=lambda_1
      settings: SourceProductName=USask Transmission Line Model Library
  Q_1 : Outport
  P_2 : Outport  Port=2
  wires:
  P_1/1 -> Tapered TLM Base/1, Sum6/1
  Q_2/1 -> Tapered TLM Base/3, Gain1/1
  Sum6/1 -> Gain2/1
  Gain2/1 -> Tapered TLM Base/2, Q_1/1
  Sum4/1 -> Tapered TLM Base/4, P_2/1
  Gain1/1 -> Sum4/2
  Tapered TLM Base/1 -> Sum6/2
  Tapered TLM Base/2 -> Sum4/1

== system usask_tlm_lib/Tapered FIR TLM Q1Q2 ==
  P_1 : Inport
  P_2 : Inport  Port=2
  Gain1 : Gain  Gain=1/Zc_2
  Gain2 : Gain  Gain=1/Zc_1
  Sum4 : Sum  Inputs=-+|
  Sum6 : Sum  Inputs=-+|
  Tapered TLM Base : usask_tlm_lib/Internal Blocks/Tapered TLM Base  Zc_1=Zc_1  Zc_2=Zc_2  beta=beta  T=T  lambda_1=lambda_1
      settings: SourceProductName=USask Transmission Line Model Library
  Q_1 : Outport
  Q_2 : Outport  Port=2
  wires:
  P_1/1 -> Sum6/2, Tapered TLM Base/1
  Sum6/1 -> Gain2/1
  Gain2/1 -> Tapered TLM Base/2, Q_1/1
  P_2/1 -> Sum4/2, Tapered TLM Base/4
  Tapered TLM Base/1 -> Sum6/1
  Tapered TLM Base/2 -> Sum4/1
  Sum4/1 -> Gain1/1
  Gain1/1 -> Tapered TLM Base/3, Q_2/1

== system usask_tlm_lib/Tapered TLM P1P2 ==
  Q_1 : Inport
  Q_2 : Inport  Port=2
  "  Delay_2 " : Subsystem
      mask Display: disp('\fontname{Times New Roman}\ite^{-j\omegaT}', 'texmode', 'on')
  "Delay_1 " : Subsystem
      mask Display: disp('\fontname{Times New Roman}\ite^{-j\omegaT}', 'texmode', 'on')
  E_1 : Subsystem
      mask Display: disp('\fontname{Times New Roman}\fontsize{30}\itE', 'texmode', 'on')
  E_2 : Subsystem
      mask Display: disp('\fontname{Times New Roman}\fontsize{30}\itE', 'texmode', 'on')
  F_1 : Subsystem
      mask Display: disp('\fontname{Times New Roman}\fontsize{30}\itF', 'texmode', 'on')
  F_2 : Subsystem
      mask Display: disp('\fontname{Times New Roman}\fontsize{30}\itF', 'texmode', 'on')
  G_1 : Subsystem
      mask Display: disp('\fontname{Times New Roman}\fontsize{30}\itG', 'texmode', 'on')
  G_2 : Subsystem
      mask Display: disp('\fontname{Times New Roman}\fontsize{30}\itG', 'texmode', 'on')
  Gain1 : Gain  Gain=Z_c
  Gain2 : Gain  Gain=Z_c
  Sum : Sum  Inputs=|++
  Sum1 : Sum  Inputs=|++
  Sum2 : Sum  Inputs=++|
  Sum3 : Sum  Inputs=++|
  Sum4 : Sum  Inputs=|++
  Sum5 : Sum  Inputs=++|
  P_1 : Outport
  P_2 : Outport  Port=2
  wires:
  Sum5/1 -> Sum3/2, P_2/1
  Gain2/1 -> Sum5/2
  Sum1/1 -> Sum5/1
  F_1/1(Out1) -> Sum/2
  Gain1/1 -> Sum4/1
  Q_2/1 -> E_2/1(Q_2), F_2/2(Q_2), Gain2/1
  "  Delay_2 "/1(delay) -> Sum2/2
  "Delay_1 "/1(delay) -> Sum1/1
  Sum2/1 -> Sum4/2
  F_2/1(F) -> Sum3/1
  Sum3/1 -> G_2/1(F + P_2)
  Sum4/1 -> Sum/1, P_1/1
  Q_1/1 -> E_1/1(Q_1), F_1/1(Q_1), Gain1/1
  G_2/1(G) -> "  Delay_2 "/1(G)
  E_1/1(E) -> Sum2/1, F_1/2(E)
  E_2/1(E) -> F_2/1(E), Sum1/2
  G_1/1(G) -> "Delay_1 "/1(G)
  Sum/1 -> G_1/1(F + P_1)

== system usask_tlm_lib/Tapered TLM P1Q2 ==
  Q_1 : Inport
  P_2 : Inport  Port=2
  "  Delay_2 " : Subsystem
      mask Display: disp('\fontname{Times New Roman}\ite^{-j\omegaT}', 'texmode', 'on')
  "Delay_1 " : Subsystem
      mask Display: disp('\fontname{Times New Roman}\ite^{-j\omegaT}', 'texmode', 'on')
  E_1 : Subsystem
      mask Display: disp('\fontname{Times New Roman}\fontsize{30}\itE', 'texmode', 'on')
  E_2 : Subsystem
      mask Display: disp('\fontname{Times New Roman}\fontsize{30}\itE', 'texmode', 'on')
  F_1 : Subsystem
      mask Display: disp('\fontname{Times New Roman}\fontsize{30}\itF', 'texmode', 'on')
  F_2 : Subsystem
      mask Display: disp('\fontname{Times New Roman}\fontsize{30}\itF', 'texmode', 'on')
  G_1 : Subsystem
      mask Display: disp('\fontname{Times New Roman}\fontsize{30}\itG', 'texmode', 'on')
  G_2 : Subsystem
      mask Display: disp('\fontname{Times New Roman}\fontsize{30}\itG', 'texmode', 'on')
  Gain1 : Gain  Gain=Z_c
  Gain3 : Gain  Gain=1/Z_c
  Sum : Sum  Inputs=|++
  Sum1 : Sum  Inputs=|++
  Sum2 : Sum  Inputs=++|
  Sum3 : Sum  Inputs=++|
  Sum4 : Sum  Inputs=|++
  Sum5 : Sum  Inputs=-+|
  P_1 : Outport
  Q_2 : Outport  Port=2
  wires:
  F_1/1(F) -> Sum/2
  Sum5/1 -> Gain3/1
  Gain1/1 -> Sum4/1
  Gain3/1 -> Q_2/1, E_2/1(Q_2), F_2/2(Q_2)
  "  Delay_2 "/1(delay) -> Sum2/2
  "Delay_1 "/1(delay) -> Sum1/1
  P_2/1 -> Sum3/2, Sum5/2
  Sum1/1 -> Sum5/1
  Sum2/1 -> Sum4/2
  F_2/1(Out1) -> Sum3/1
  Sum3/1 -> G_2/1(F + P_2)
  Sum4/1 -> Sum/1, P_1/1
  Q_1/1 -> E_1/1(Q_1), F_1/1(Q_1), Gain1/1
  G_2/1(G) -> "  Delay_2 "/1(G)
  E_1/1(E) -> Sum2/1, F_1/2(E)
  E_2/1(E) -> F_2/1(E), Sum1/2
  G_1/1(G) -> "Delay_1 "/1(G)
  Sum/1 -> G_1/1(F + P_1)

== system usask_tlm_lib/Tapered TLM Q1P2 ==
  P_1 : Inport
  Q_2 : Inport  Port=2
  "  Delay_2 " : Subsystem
      mask Display: disp('\fontname{Times New Roman}\ite^{-j\omegaT}', 'texmode', 'on')
  "Delay_1 " : Subsystem
      mask Display: disp('\fontname{Times New Roman}\ite^{-j\omegaT}', 'texmode', 'on')
  E_1 : Subsystem
      mask Display: disp('\fontname{Times New Roman}\fontsize{30}\itE', 'texmode', 'on')
  E_2 : Subsystem
      mask Display: disp('\fontname{Times New Roman}\fontsize{30}\itE', 'texmode', 'on')
  F_1 : Subsystem
      mask Display: disp('\fontname{Times New Roman}\fontsize{30}\itF', 'texmode', 'on')
  F_2 : Subsystem
      mask Display: disp('\fontname{Times New Roman}\fontsize{30}\itF', 'texmode', 'on')
  G_1 : Subsystem
      mask Display: disp('\fontname{Times New Roman}\fontsize{30}\itG', 'texmode', 'on')
  G_2 : Subsystem
      mask Display: disp('\fontname{Times New Roman}\fontsize{30}\itG', 'texmode', 'on')
  Gain1 : Gain  Gain=Z_c
  Gain2 : Gain  Gain=1/Z_c
  Sum : Sum  Inputs=|++
  Sum1 : Sum  Inputs=|++
  Sum2 : Sum  Inputs=++|
  Sum3 : Sum  Inputs=++|
  Sum4 : Sum  Inputs=++|
  Sum6 : Sum  Inputs=|+-
  Q_1 : Outport
  P_2 : Outport  Port=2
  wires:
  Gain1/1 -> Sum4/2
  Sum4/1 -> Sum3/2, P_2/1
  Sum1/1 -> Sum4/1
  Sum2/1 -> Sum6/2
  Gain2/1 -> E_1/1(Q_1), F_1/1(Q_1), Q_1/1
  Sum6/1 -> Gain2/1
  F_1/1(F) -> Sum/2
  Q_2/1 -> E_2/1(Q_2), F_2/2(Q_2), Gain1/1
  "  Delay_2 "/1(delay) -> Sum2/2
  "Delay_1 "/1(delay) -> Sum1/1
  F_2/1(Out1) -> Sum3/1
  Sum3/1 -> G_2/1(F + P_2)
  P_1/1 -> Sum/1, Sum6/1
  G_2/1(G) -> "  Delay_2 "/1(G)
  E_1/1(E) -> Sum2/1, F_1/2(E)
  E_2/1(E) -> F_2/1(E), Sum1/2
  G_1/1(G) -> "Delay_1 "/1(G)
  Sum/1 -> G_1/1(F + P_1)

== system usask_tlm_lib/Tapered TLM Q1Q2 ==
  P_1 : Inport
  P_2 : Inport  Port=2
  "  Delay_2 " : Subsystem
      mask Display: disp('\fontname{Times New Roman}\ite^{-j\omegaT}', 'texmode', 'on')
  "Delay_1 " : Subsystem
      mask Display: disp('\fontname{Times New Roman}\ite^{-j\omegaT}', 'texmode', 'on')
  E_1 : Subsystem
      mask Display: disp('\fontname{Times New Roman}\fontsize{30}\itE', 'texmode', 'on')
  E_2 : Subsystem
      mask Display: disp('\fontname{Times New Roman}\fontsize{30}\itE', 'texmode', 'on')
  F_1 : Subsystem
      mask Display: disp('\fontname{Times New Roman}\fontsize{30}\itF', 'texmode', 'on')
  F_2 : Subsystem
      mask Display: disp('\fontname{Times New Roman}\fontsize{30}\itF', 'texmode', 'on')
  G_1 : Subsystem
      mask Display: disp('\fontname{Times New Roman}\fontsize{30}\itG', 'texmode', 'on')
  G_2 : Subsystem
      mask Display: disp('\fontname{Times New Roman}\fontsize{30}\itG', 'texmode', 'on')
  Gain2 : Gain  Gain=1/Z_c
  Gain3 : Gain  Gain=1/Z_c
  Sum : Sum  Inputs=|++
  Sum1 : Sum  Inputs=|++
  Sum2 : Sum  Inputs=++|
  Sum3 : Sum  Inputs=++|
  Sum5 : Sum  Inputs=-+|
  Sum6 : Sum  Inputs=|+-
  Q_1 : Outport
  Q_2 : Outport  Port=2
  wires:
  Sum2/1 -> Sum6/2
  Gain2/1 -> E_1/1(Q_1), F_1/1(Q_1), Q_1/1
  Sum6/1 -> Gain2/1
  P_1/1 -> Sum/1, Sum6/1
  F_1/1(F) -> Sum/2
  Sum5/1 -> Gain3/1
  Gain3/1 -> Q_2/1, E_2/1(Q_2), F_2/2(Q_2)
  "  Delay_2 "/1(delay) -> Sum2/2
  "Delay_1 "/1(delay) -> Sum1/1
  P_2/1 -> Sum3/2, Sum5/2
  Sum1/1 -> Sum5/1
  F_2/1(F) -> Sum3/1
  Sum3/1 -> G_2/1(F + P_2)
  G_2/1(G) -> "  Delay_2 "/1(G)
  E_1/1(E) -> Sum2/1, F_1/2(E)
  E_2/1(E) -> F_2/1(E), Sum1/2
  G_1/1(G) -> "Delay_1 "/1(G)
  Sum/1 -> G_1/1(F + P_1)

== system usask_tlm_lib/Elastic TLM P1P2/  Delay_2  ==
  G : Inport
  Transport Delay : TransportDelay  DelayTime=T_prime
  delay : Outport
  wires:
  G/1 -> Transport Delay/1
  Transport Delay/1 -> delay/1

== system usask_tlm_lib/Elastic TLM P1P2/Delay_1  ==
  G : Inport
  Transport Delay : TransportDelay  DelayTime=T_prime
  delay : Outport
  wires:
  G/1 -> Transport Delay/1
  Transport Delay/1 -> delay/1

== system usask_tlm_lib/Elastic TLM P1P2/E_1 ==
  note: Equation (14) from ven der Buhs et al. 2017
  Q_1 : Inport
  Gain : Gain  Gain=Z_c
  Sum : Sum  Inputs=++++++
  k = 1 : TransferFcn  Numerator=[m_E(1)]  Denominator=[T n(1)]
  k = 2 : TransferFcn  Numerator=[m_E(2)]  Denominator=[T n(2)]
  k = 3 : TransferFcn  Numerator=[m_E(3)]  Denominator=[T n(3)]
  k = 4 : TransferFcn  Numerator=[m_E(4)]  Denominator=[T n(4)]
  k = 5 : TransferFcn  Numerator=[m_E(5)]  Denominator=[T n(5)]
  k = 6 : TransferFcn  Numerator=[m_E(6)]  Denominator=[T n(6)]
  E : Outport
  wires:
  Gain/1 -> E/1
  Sum/1 -> Gain/1
  k = 1/1 -> Sum/1
  k = 2/1 -> Sum/2
  k = 3/1 -> Sum/3
  k = 4/1 -> Sum/4
  k = 5/1 -> Sum/5
  k = 6/1 -> Sum/6
  Q_1/1 -> k = 2/1, k = 1/1, k = 3/1, k = 6/1, k = 5/1, k = 4/1

== system usask_tlm_lib/Elastic TLM P1P2/E_2 ==
  note: Equation (14) from ven der Buhs et al. 2017
  Q_2 : Inport
  Gain : Gain  Gain=Z_c
  Sum : Sum  Inputs=++++++
  k = 1 : TransferFcn  Numerator=[m_E(1)]  Denominator=[T n(1)]
  k = 2 : TransferFcn  Numerator=[m_E(2)]  Denominator=[T n(2)]
  k = 3 : TransferFcn  Numerator=[m_E(3)]  Denominator=[T n(3)]
  k = 4 : TransferFcn  Numerator=[m_E(4)]  Denominator=[T n(4)]
  k = 5 : TransferFcn  Numerator=[m_E(5)]  Denominator=[T n(5)]
  k = 6 : TransferFcn  Numerator=[m_E(6)]  Denominator=[T n(6)]
  E : Outport
  wires:
  Gain/1 -> E/1
  Sum/1 -> Gain/1
  k = 1/1 -> Sum/1
  k = 2/1 -> Sum/2
  k = 3/1 -> Sum/3
  k = 4/1 -> Sum/4
  k = 5/1 -> Sum/5
  k = 6/1 -> Sum/6
  Q_2/1 -> k = 2/1, k = 1/1, k = 3/1, k = 6/1, k = 5/1, k = 4/1

== system usask_tlm_lib/Elastic TLM P1P2/F_1 ==
  note: Equation (15) from ven der Buhs et al. 2017
  Q_1 : Inport
  E : Inport  Port=2
  Gain : Gain  Gain=b
  Gain1 : Gain  Gain=Z_c
  Sum : Sum
  Out1 : Outport
  wires:
  Gain/1 -> Sum/2
  Gain1/1 -> Sum/1
  Sum/1 -> Out1/1
  Q_1/1 -> Gain1/1
  E/1 -> Gain/1

== system usask_tlm_lib/Elastic TLM P1P2/F_2 ==
  note: Equation (15) from ven der Buhs et al. 2017
  E : Inport
  Q_2 : Inport  Port=2
  Gain : Gain  Gain=b
  Gain1 : Gain  Gain=Z_c
  Sum : Sum
  F : Outport
  wires:
  E/1 -> Gain/1
  Q_2/1 -> Gain1/1
  Sum/1 -> F/1
  Gain1/1 -> Sum/1
  Gain/1 -> Sum/2

== system usask_tlm_lib/Elastic TLM P1P2/G_1 ==
  note: Equation (17) from ven der Buhs et al. 2017
  F + P_1 : Inport
  Sum : Sum  Inputs=+------
  k = 1 : TransferFcn  Numerator=[m_G(1)*T 0]  Denominator=[T n(1)]
  k = 2 : TransferFcn  Numerator=[m_G(2)*T 0]  Denominator=[T n(2)]
  k = 3 : TransferFcn  Numerator=[m_G(3)*T 0]  Denominator=[T n(3)]
  k = 4 : TransferFcn  Numerator=[m_G(4)*T 0]  Denominator=[T n(4)]
  k = 5 : TransferFcn  Numerator=[m_G(5)*T 0]  Denominator=[T n(5)]
  k = 6 : TransferFcn  Numerator=[m_G(6)*T 0]  Denominator=[T n(6)]
  G : Outport
  wires:
  Sum/1 -> G/1
  F + P_1/1 -> k = 4/1, k = 6/1, k = 5/1, k = 1/1, Sum/1, k = 2/1, k = 3/1
  k = 3/1 -> Sum/4
  k = 1/1 -> Sum/2
  k = 2/1 -> Sum/3
  k = 4/1 -> Sum/5
  k = 5/1 -> Sum/6
  k = 6/1 -> Sum/7

== system usask_tlm_lib/Elastic TLM P1P2/G_2 ==
  note: Equation (17) from ven der Buhs et al. 2017
  F + P_2 : Inport
  Sum : Sum  Inputs=+------
  k = 1 : TransferFcn  Numerator=[m_G(1)*T 0]  Denominator=[T n(1)]
  k = 2 : TransferFcn  Numerator=[m_G(2)*T 0]  Denominator=[T n(2)]
  k = 3 : TransferFcn  Numerator=[m_G(3)*T 0]  Denominator=[T n(3)]
  k = 4 : TransferFcn  Numerator=[m_G(4)*T 0]  Denominator=[T n(4)]
  k = 5 : TransferFcn  Numerator=[m_G(5)*T 0]  Denominator=[T n(5)]
  k = 6 : TransferFcn  Numerator=[m_G(6)*T 0]  Denominator=[T n(6)]
  G : Outport
  wires:
  Sum/1 -> G/1
  F + P_2/1 -> k = 4/1, k = 6/1, k = 5/1, k = 1/1, Sum/1, k = 2/1, k = 3/1
  k = 3/1 -> Sum/4
  k = 1/1 -> Sum/2
  k = 2/1 -> Sum/3
  k = 4/1 -> Sum/5
  k = 5/1 -> Sum/6
  k = 6/1 -> Sum/7

== system usask_tlm_lib/Elastic TLM P1Q2/  Delay_2  ==
  G : Inport
  Transport Delay : TransportDelay  DelayTime=T_prime
  delay : Outport
  wires:
  G/1 -> Transport Delay/1
  Transport Delay/1 -> delay/1

== system usask_tlm_lib/Elastic TLM P1Q2/Delay_1  ==
  G : Inport
  Transport Delay : TransportDelay  DelayTime=T_prime
  delay : Outport
  wires:
  G/1 -> Transport Delay/1
  Transport Delay/1 -> delay/1

== system usask_tlm_lib/Elastic TLM P1Q2/E_1 ==
  note: Equation (14) from ven der Buhs et al. 2017
  Q_1 : Inport
  Gain : Gain  Gain=Z_c
  Sum : Sum  Inputs=++++++
  k = 1 : TransferFcn  Numerator=[m_E(1)]  Denominator=[T n(1)]
  k = 2 : TransferFcn  Numerator=[m_E(2)]  Denominator=[T n(2)]
  k = 3 : TransferFcn  Numerator=[m_E(3)]  Denominator=[T n(3)]
  k = 4 : TransferFcn  Numerator=[m_E(4)]  Denominator=[T n(4)]
  k = 5 : TransferFcn  Numerator=[m_E(5)]  Denominator=[T n(5)]
  k = 6 : TransferFcn  Numerator=[m_E(6)]  Denominator=[T n(6)]
  E : Outport
  wires:
  Gain/1 -> E/1
  Sum/1 -> Gain/1
  k = 1/1 -> Sum/1
  k = 2/1 -> Sum/2
  k = 3/1 -> Sum/3
  k = 4/1 -> Sum/4
  k = 5/1 -> Sum/5
  k = 6/1 -> Sum/6
  Q_1/1 -> k = 2/1, k = 1/1, k = 3/1, k = 6/1, k = 5/1, k = 4/1

== system usask_tlm_lib/Elastic TLM P1Q2/E_2 ==
  note: Equation (14) from ven der Buhs et al. 2017
  Q_2 : Inport
  Gain : Gain  Gain=Z_c
  Sum : Sum  Inputs=++++++
  k = 1 : TransferFcn  Numerator=[m_E(1)]  Denominator=[T n(1)]
  k = 2 : TransferFcn  Numerator=[m_E(2)]  Denominator=[T n(2)]
  k = 3 : TransferFcn  Numerator=[m_E(3)]  Denominator=[T n(3)]
  k = 4 : TransferFcn  Numerator=[m_E(4)]  Denominator=[T n(4)]
  k = 5 : TransferFcn  Numerator=[m_E(5)]  Denominator=[T n(5)]
  k = 6 : TransferFcn  Numerator=[m_E(6)]  Denominator=[T n(6)]
  E : Outport
  wires:
  Gain/1 -> E/1
  Sum/1 -> Gain/1
  k = 1/1 -> Sum/1
  k = 2/1 -> Sum/2
  k = 3/1 -> Sum/3
  k = 4/1 -> Sum/4
  k = 5/1 -> Sum/5
  k = 6/1 -> Sum/6
  Q_2/1 -> k = 2/1, k = 1/1, k = 3/1, k = 6/1, k = 5/1, k = 4/1

== system usask_tlm_lib/Elastic TLM P1Q2/F_1 ==
  note: Equation (15) from ven der Buhs et al. 2017
  Q_1 : Inport
  E : Inport  Port=2
  Gain : Gain  Gain=b
  Gain1 : Gain  Gain=Z_c
  Sum : Sum
  F : Outport
  wires:
  Gain/1 -> Sum/2
  Gain1/1 -> Sum/1
  Sum/1 -> F/1
  Q_1/1 -> Gain1/1
  E/1 -> Gain/1

== system usask_tlm_lib/Elastic TLM P1Q2/F_2 ==
  note: Equation (15) from ven der Buhs et al. 2017
  E : Inport
  Q_2 : Inport  Port=2
  Gain : Gain  Gain=b
  Gain1 : Gain  Gain=Z_c
  Sum : Sum
  Out1 : Outport
  wires:
  E/1 -> Gain/1
  Q_2/1 -> Gain1/1
  Sum/1 -> Out1/1
  Gain1/1 -> Sum/1
  Gain/1 -> Sum/2

== system usask_tlm_lib/Elastic TLM P1Q2/G_1 ==
  note: Equation (17) from ven der Buhs et al. 2017
  F + P_1 : Inport
  Sum : Sum  Inputs=+------
  k = 1 : TransferFcn  Numerator=[m_G(1)*T 0]  Denominator=[T n(1)]
  k = 2 : TransferFcn  Numerator=[m_G(2)*T 0]  Denominator=[T n(2)]
  k = 3 : TransferFcn  Numerator=[m_G(3)*T 0]  Denominator=[T n(3)]
  k = 4 : TransferFcn  Numerator=[m_G(4)*T 0]  Denominator=[T n(4)]
  k = 5 : TransferFcn  Numerator=[m_G(5)*T 0]  Denominator=[T n(5)]
  k = 6 : TransferFcn  Numerator=[m_G(6)*T 0]  Denominator=[T n(6)]
  G : Outport
  wires:
  Sum/1 -> G/1
  F + P_1/1 -> k = 4/1, k = 6/1, k = 5/1, k = 1/1, Sum/1, k = 2/1, k = 3/1
  k = 3/1 -> Sum/4
  k = 1/1 -> Sum/2
  k = 2/1 -> Sum/3
  k = 4/1 -> Sum/5
  k = 5/1 -> Sum/6
  k = 6/1 -> Sum/7

== system usask_tlm_lib/Elastic TLM P1Q2/G_2 ==
  note: Equation (17) from ven der Buhs et al. 2017
  F + P_2 : Inport
  Sum : Sum  Inputs=+------
  k = 1 : TransferFcn  Numerator=[m_G(1)*T 0]  Denominator=[T n(1)]
  k = 2 : TransferFcn  Numerator=[m_G(2)*T 0]  Denominator=[T n(2)]
  k = 3 : TransferFcn  Numerator=[m_G(3)*T 0]  Denominator=[T n(3)]
  k = 4 : TransferFcn  Numerator=[m_G(4)*T 0]  Denominator=[T n(4)]
  k = 5 : TransferFcn  Numerator=[m_G(5)*T 0]  Denominator=[T n(5)]
  k = 6 : TransferFcn  Numerator=[m_G(6)*T 0]  Denominator=[T n(6)]
  G : Outport
  wires:
  Sum/1 -> G/1
  F + P_2/1 -> k = 4/1, k = 6/1, k = 5/1, k = 1/1, Sum/1, k = 2/1, k = 3/1
  k = 3/1 -> Sum/4
  k = 1/1 -> Sum/2
  k = 2/1 -> Sum/3
  k = 4/1 -> Sum/5
  k = 5/1 -> Sum/6
  k = 6/1 -> Sum/7

== system usask_tlm_lib/Elastic TLM Q1P2/  Delay_2  ==
  G : Inport
  Transport Delay : TransportDelay  DelayTime=T_prime
  delay : Outport
  wires:
  G/1 -> Transport Delay/1
  Transport Delay/1 -> delay/1

== system usask_tlm_lib/Elastic TLM Q1P2/Delay_1  ==
  G : Inport
  Transport Delay : TransportDelay  DelayTime=T_prime
  delay : Outport
  wires:
  G/1 -> Transport Delay/1
  Transport Delay/1 -> delay/1

== system usask_tlm_lib/Elastic TLM Q1P2/E_1 ==
  note: Equation (14) from ven der Buhs et al. 2017
  Q_1 : Inport
  Gain : Gain  Gain=Z_c
  Sum : Sum  Inputs=++++++
  k = 1 : TransferFcn  Numerator=[m_E(1)]  Denominator=[T n(1)]
  k = 2 : TransferFcn  Numerator=[m_E(2)]  Denominator=[T n(2)]
  k = 3 : TransferFcn  Numerator=[m_E(3)]  Denominator=[T n(3)]
  k = 4 : TransferFcn  Numerator=[m_E(4)]  Denominator=[T n(4)]
  k = 5 : TransferFcn  Numerator=[m_E(5)]  Denominator=[T n(5)]
  k = 6 : TransferFcn  Numerator=[m_E(6)]  Denominator=[T n(6)]
  E : Outport
  wires:
  Gain/1 -> E/1
  Sum/1 -> Gain/1
  k = 1/1 -> Sum/1
  k = 2/1 -> Sum/2
  k = 3/1 -> Sum/3
  k = 4/1 -> Sum/4
  k = 5/1 -> Sum/5
  k = 6/1 -> Sum/6
  Q_1/1 -> k = 2/1, k = 1/1, k = 3/1, k = 6/1, k = 5/1, k = 4/1

== system usask_tlm_lib/Elastic TLM Q1P2/E_2 ==
  note: Equation (14) from ven der Buhs et al. 2017
  Q_2 : Inport
  Gain : Gain  Gain=Z_c
  Sum : Sum  Inputs=++++++
  k = 1 : TransferFcn  Numerator=[m_E(1)]  Denominator=[T n(1)]
  k = 2 : TransferFcn  Numerator=[m_E(2)]  Denominator=[T n(2)]
  k = 3 : TransferFcn  Numerator=[m_E(3)]  Denominator=[T n(3)]
  k = 4 : TransferFcn  Numerator=[m_E(4)]  Denominator=[T n(4)]
  k = 5 : TransferFcn  Numerator=[m_E(5)]  Denominator=[T n(5)]
  k = 6 : TransferFcn  Numerator=[m_E(6)]  Denominator=[T n(6)]
  E : Outport
  wires:
  Gain/1 -> E/1
  Sum/1 -> Gain/1
  k = 1/1 -> Sum/1
  k = 2/1 -> Sum/2
  k = 3/1 -> Sum/3
  k = 4/1 -> Sum/4
  k = 5/1 -> Sum/5
  k = 6/1 -> Sum/6
  Q_2/1 -> k = 2/1, k = 1/1, k = 3/1, k = 6/1, k = 5/1, k = 4/1

== system usask_tlm_lib/Elastic TLM Q1P2/F_1 ==
  note: Equation (15) from ven der Buhs et al. 2017
  Q_1 : Inport
  E : Inport  Port=2
  Gain : Gain  Gain=b
  Gain1 : Gain  Gain=Z_c
  Sum : Sum
  F : Outport
  wires:
  Gain/1 -> Sum/2
  Gain1/1 -> Sum/1
  Sum/1 -> F/1
  Q_1/1 -> Gain1/1
  E/1 -> Gain/1

== system usask_tlm_lib/Elastic TLM Q1P2/F_2 ==
  note: Equation (15) from ven der Buhs et al. 2017
  E : Inport
  Q_2 : Inport  Port=2
  Gain : Gain  Gain=b
  Gain1 : Gain  Gain=Z_c
  Sum : Sum
  Out1 : Outport
  wires:
  E/1 -> Gain/1
  Q_2/1 -> Gain1/1
  Sum/1 -> Out1/1
  Gain1/1 -> Sum/1
  Gain/1 -> Sum/2
